simulink model "PNG_guidanceloop_modified"  (R2020a)
settings: Solver=VariableStepAuto  StartTime=0.0  StopTime=10  RelTol=1e-3
values from neighbouring files (symbols this model uses):
  coeffs_den = double(fliplr(coeffs(eq_den,s)))    [errSlxParas.m]
  coeffs_num = [double(fliplr(coeffs(eq_num,s))) 0]    [errSlxParas.m]
  Tf_Tg = 15    [errSlxParas.m]
settings Model: OrderedModelArguments=off  Creator=anwaei  LastModifiedBy=anwaei

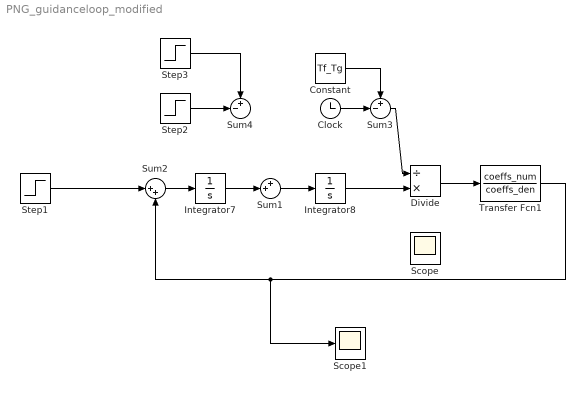
== system PNG_guidanceloop_modified ==
  Clock : Clock
  Constant : Constant  Value=Tf_Tg
  Divide : Product  Inputs=/*
  Integrator7 : Integrator
  Integrator8 : Integrator
  Scope : Scope
  Scope1 : Scope
  Step1 : Step  SampleTime=0
  Step2 : Step  Time=1.5  SampleTime=0
  Step3 : Step  SampleTime=0
  Sum1 : Sum  Inputs=++|
  Sum2 : Sum  Inputs=|++
  Sum3 : Sum  Inputs=+-|
  Sum4 : Sum  Inputs=+-|
  Transfer Fcn1 : TransferFcn  Numerator=coeffs_num  Denominator=coeffs_den
  wires:
  Transfer Fcn1/1 -> Scope1/1, Sum2/2
  Integrator7/1 -> Sum1/2
  Sum1/1 -> Integrator8/1
  Step1/1 -> Sum2/1
  Constant/1 -> Sum3/1
  Clock/1 -> Sum3/2
  Sum3/1 -> Divide/1
  Divide/1 -> Transfer Fcn1/1
  Step2/1 -> Sum4/2
  Step3/1 -> Sum4/1
  Sum2/1 -> Integrator7/1
  Integrator8/1 -> Divide/2
